simulink model "project_01_model"  (R2023b)
settings: Solver=VariableStepAuto  StartTime=0.0  StopTime=20  RelTol=1e-3
values from neighbouring files (symbols this model uses):
  A = jacobian(x_dot, x)    [cube_ctrl.m]    (also in cube_ctrl_sim.m; project_01_script.m = [0 1 0 0)
  alpha = 0.5    [project_01_script.m]
  B = jacobian(x_dot, u)    [cube_ctrl.m]    (also in cube_ctrl_sim.m; project_01_script.m = [0)
  C = zeros(2,10)    [cube_ctrl.m]    (also in cube_ctrl_sim.m; project_01_script.m = [1 0 0 0)
  D = zeros(2,3)    [cube_ctrl.m]    (also in cube_ctrl_sim.m; project_01_script.m = [0;0])
  K = [Ka(2) Ka(3) Ka(4) Ka(5)]    [project_01_script.m]
  Ki = Ka(1)    [project_01_script.m]
  L = place(A', C', Po)'    [project_01_script.m]
settings Model: Creator=charl  LastModifiedBy=charl

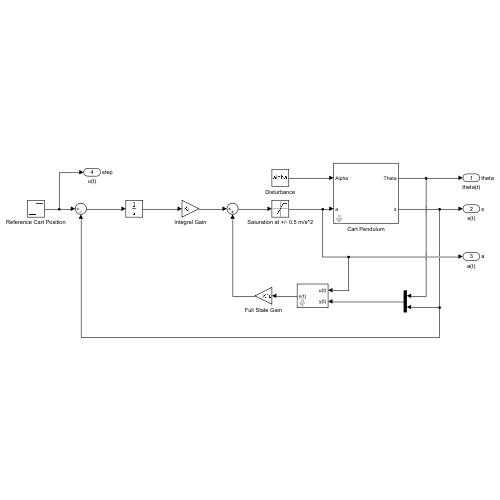
[thumbnail: Simulink's stored preview of the top-level diagram]
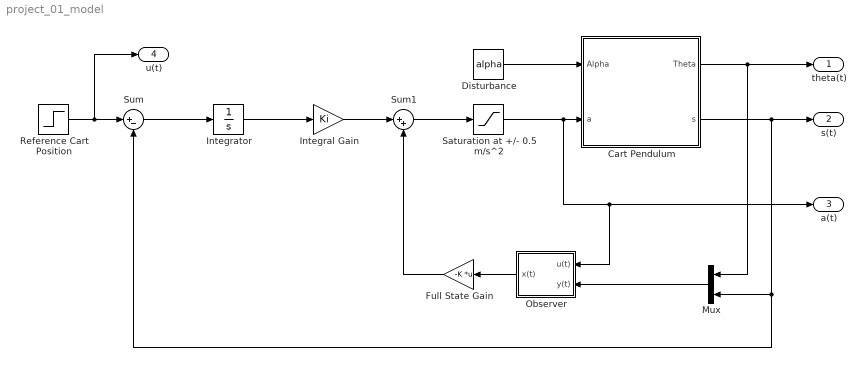
== system project_01_model ==
  Cart Pendulum : Subsystem  mask{l=0.5, g=9.8}
      mask prompts: l "Length of Pendulum"; g "Gravity"
  Disturbance : Constant  Value=alpha
  Full State Gain : Gain  Gain=-K  Multiplication=Matrix(K*u)
  Integral Gain : Gain  Gain=Ki
  Integrator : Integrator
  Mux : Mux  Inputs=2
  Observer : Subsystem  mask{A=A, B=B, C=C, D=D, L=L}
      mask prompts: A "System Matrix"; B "Control Vector"; C "Output Matrix"; D "Transmission Vector"; L "Observer Gain Matrix"
  Reference Cart Position : Step  Time=0  SampleTime=0
  Saturation at +/- 0.5 m/s^2 : Saturate
  Sum : Sum  Inputs=|+-
  Sum1 : Sum  Inputs=|++
  theta(t) : Outport  SignalName=theta
  s(t) : Outport  Port=2  SignalName=s
  a(t) : Outport  Port=3  SignalName=a
  u(t) : Outport  Port=4  SignalName=step
  wires:
  Reference Cart Position/1 -> u(t)/1, Sum/1
  Sum/1 -> Integrator/1
  Integrator/1 -> Integral Gain/1
  Disturbance/1 -> Cart Pendulum/1(Alpha)
  Cart Pendulum/1(Theta) -> Mux/1, theta(t)/1
  Cart Pendulum/2(s) -> Sum/2, Mux/2, s(t)/1
  Saturation at +/- 0.5 m/s^2/1 -> Observer/1(u(t)), a(t)/1, Cart Pendulum/2(a)
  Mux/1 -> Observer/2(y(t))
  Observer/1(x(t)) -> Full State Gain/1
  Sum1/1 -> Saturation at +/- 0.5 m/s^2/1
  Integral Gain/1 -> Sum1/1
  Full State Gain/1 -> Sum1/2

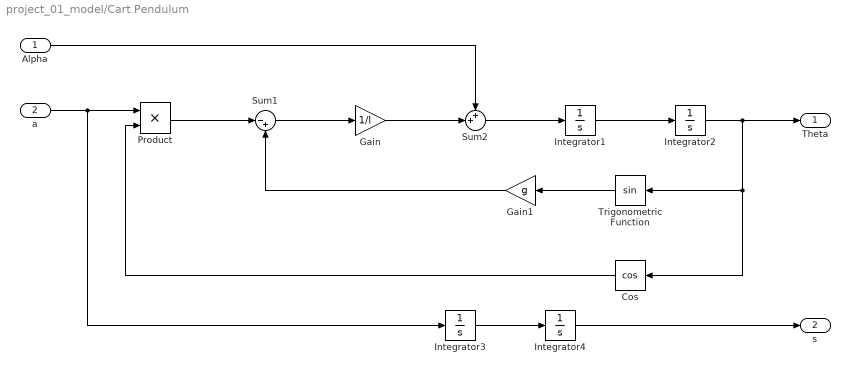
== system project_01_model/Cart Pendulum ==
  Alpha : Inport
  a : Inport  Port=2
  Cos : Trigonometry  Operator=cos
  Gain : Gain  Gain=1/l
  Gain1 : Gain  Gain=g
  Integrator{1..4} (4 alike) : Integrator
  Product : Product
  Sum1 : Sum  Inputs=|-+
  Sum2 : Sum  Inputs=++|
  Trigonometric Function : Trigonometry
  Theta : Outport
  s : Outport  Port=2
  wires:
  Integrator2/1 -> Theta/1, Cos/1, Trigonometric Function/1
  a/1 -> Integrator3/1, Product/1
  Integrator1/1 -> Integrator2/1
  Integrator4/1 -> s/1
  Integrator3/1 -> Integrator4/1
  Sum2/1 -> Integrator1/1
  Product/1 -> Sum1/1
  Gain/1 -> Sum2/2
  Gain1/1 -> Sum1/2
  Sum1/1 -> Gain/1
  Cos/1 -> Product/2
  Trigonometric Function/1 -> Gain1/1
  Alpha/1 -> Sum2/1

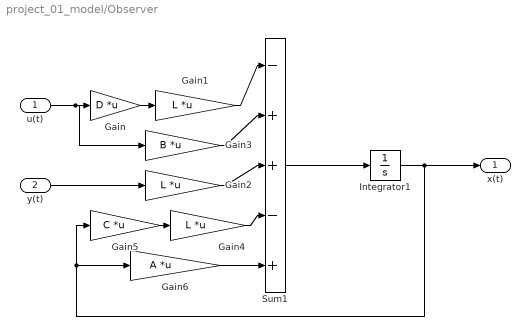
== system project_01_model/Observer ==
  u(t) : Inport
  y(t) : Inport  Port=2
  Gain : Gain  Gain=D  Multiplication=Matrix(K*u)
  Gain1 : Gain  Gain=L  Multiplication=Matrix(K*u) (u vector)
  Gain2 : Gain  Gain=L  Multiplication=Matrix(K*u) (u vector)
  Gain3 : Gain  Gain=B  Multiplication=Matrix(K*u)
  Gain4 : Gain  Gain=L  Multiplication=Matrix(K*u) (u vector)
  Gain5 : Gain  Gain=C  Multiplication=Matrix(K*u) (u vector)
  Gain6 : Gain  Gain=A  Multiplication=Matrix(K*u) (u vector)
  Integrator1 : Integrator
  Sum1 : Sum  Inputs=|-++-+
  x(t) : Outport
  wires:
  Integrator1/1 -> x(t)/1, Gain5/1, Gain6/1
  Gain4/1 -> Sum1/4
  Gain6/1 -> Sum1/5
  y(t)/1 -> Gain2/1
  u(t)/1 -> Gain3/1, Gain/1
  Gain5/1 -> Gain4/1
  Gain1/1 -> Sum1/1
  Gain2/1 -> Sum1/3
  Gain/1 -> Gain1/1
  Gain3/1 -> Sum1/2
  Sum1/1 -> Integrator1/1
